simulink model "sampleModel2013"  (R2023a)
settings: Solver=VariableStepAuto  StartTime=0.0  StopTime=10.0  RelTol=1e-3
libraries: hdlsllib x3, simulink x1
settings Model: Creator=user1  LastModifiedBy=user1

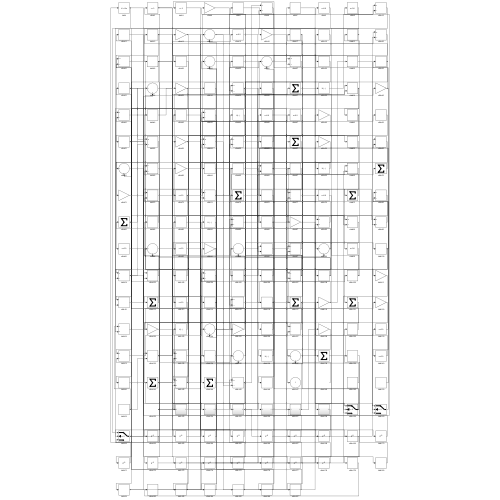
[thumbnail: Simulink's stored preview of the top-level diagram]
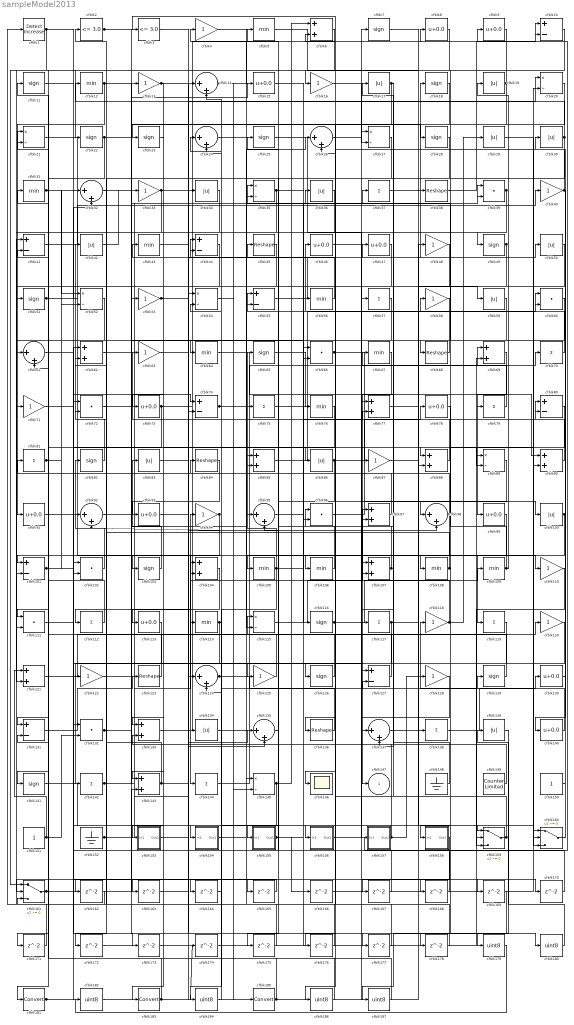
== system sampleModel2013 ==
  cfblk1 : simulink/Logic and Bit Operations/Detect Increase  vinit=0.0  OutDataTypeStr=boolean
      settings: LibrarySourceBlock=|
      | hdlsllib/Logic and Bit
      | Operations/Detect
      | Increase
  cfblk{10,41,44,55,74,80,101,127,131} (9 alike) : Sum  Inputs=+-
  cfblk{17,19,29..30,34,36,42,50,59,83,86,100,134,139} (14 alike) : Abs  SaturateOnIntegerOverflow=off
  cfblk{39,60,66,72,96,102,111,132} (8 alike) : DotProduct  OutDataTypeStr=Inherit: Inherit via internal rule
  cfblk{7,11,18,22..23,25,28,49,51,65,82,103,116,126,129,141} (16 alike) : Signum
  cfblk{6,62,69,77,85,88,90,97,104,107,121,133,143} (13 alike) : Sum
  cfblk{5,12,31,43,56,64,67,76,105..106,108..109,114} (13 alike) : MinMax
  cfblk{4,13,16,33,40,48,53,58,63,71,87,94,110,118,120,122,125,128} (18 alike) : Gain
  cfblk{37,57,70,75,79,81,112,117,119,138,142,144} (12 alike) : Sum  Inputs=+
  cfblk{8..9,15,46..47,73,78,91,93,99,113,130,140} (13 alike) : Bias  Bias=0.0  SaturateOnIntegerOverflow=off
  cfblk{20..21,27,35,52,54,89,115,145} (9 alike) : Product  Inputs=*/  RndMeth=Zero  SaturateOnIntegerOverflow=on
  cfblk{38,45,68,84,123,136} (6 alike) : Reshape
  cfblk{14,24,26,32,61,92,95,98,124,135,137} (11 alike) : Sum  Inputs=|++
  cfblk146 : Scope
  cfblk148 : Ground
  cfblk149 : hdlsllib/Sources/Counter Limited  uplimit=7  tsamp=-1
  cfblk150 : Constant  SampleTime=-1
  cfblk151 : Constant  SampleTime=-1
  cfblk152 : Ground
  cfblk153 : Subsystem
      settings: LibrarySourceBlock=|
      | hdlsllib/Ports &
      | Subsystems/Subsystem
  cfblk154 : Subsystem
      settings: LibrarySourceBlock=|
      | hdlsllib/Ports &
      | Subsystems/Subsystem
  cfblk155 : Subsystem
      settings: LibrarySourceBlock=|
      | hdlsllib/Ports &
      | Subsystems/Subsystem
  cfblk156 : Subsystem
      settings: LibrarySourceBlock=|
      | hdlsllib/Ports &
      | Subsystems/Subsystem
  cfblk157 : Subsystem
      settings: LibrarySourceBlock=|
      | hdlsllib/Ports &
      | Subsystems/Subsystem
  cfblk158 : Subsystem
      settings: LibrarySourceBlock=|
      | hdlsllib/Ports &
      | Subsystems/Subsystem
  cfblk159 : Switch  SaturateOnIntegerOverflow=off  InputSameDT=off
  cfblk160 : Switch  SaturateOnIntegerOverflow=off  InputSameDT=off
  cfblk161 : Switch  SaturateOnIntegerOverflow=off  InputSameDT=off
  cfblk{162..178} (17 alike) : Delay  SampleTime=1
  cfblk{179..180,182,184,186..187} (6 alike) : DataTypeConversion  OutDataTypeStr=uint8  SaturateOnIntegerOverflow=off  RndMeth=Floor
  cfblk181 : DataTypeConversion  SaturateOnIntegerOverflow=off  RndMeth=Floor
  cfblk183 : DataTypeConversion  SaturateOnIntegerOverflow=off  RndMeth=Floor
  cfblk185 : DataTypeConversion  SaturateOnIntegerOverflow=off  RndMeth=Floor
  cfblk2 : hdlsllib/Logic and Bit Operations/Compare To Constant  relop=<=  const=3.0  OutDataTypeStr=boolean
  cfblk3 : hdlsllib/Logic and Bit Operations/Compare To Constant  relop=<=  const=3.0  OutDataTypeStr=boolean
  cfblk147 : Outport  VectorParamsAs1DForOutWhenUnconnected=off
  wires:
  cfblk100/1 -> cfblk119/1, cfblk30/1, cfblk160/3
  cfblk42/1 -> cfblk33/1
  cfblk86/1 -> cfblk78/1, cfblk125/1
  cfblk160/1 -> cfblk80/1
  cfblk70/1 -> cfblk46/1
  cfblk141/1 -> cfblk156/1(In1)
  cfblk12/1 -> cfblk91/1, cfblk89/1
  cfblk73/1 -> cfblk45/1, cfblk101/1
  cfblk96/1 -> cfblk98/1
  cfblk140/1 -> cfblk118/1
  cfblk112/1 -> cfblk31/1
  cfblk142/1 -> cfblk37/1, cfblk120/1
  cfblk64/1 -> cfblk90/1
  cfblk135/1 -> cfblk5/1
  cfblk41/1 -> cfblk40/1
  cfblk144/1 -> cfblk69/1
  cfblk81/1 -> cfblk11/1, cfblk52/2
  cfblk40/1 -> cfblk3/1, cfblk140/1
  cfblk131/1 -> cfblk123/1
  cfblk55/1 -> cfblk18/1
  cfblk35/1 -> cfblk111/1, cfblk89/2
  cfblk66/1 -> cfblk100/1, cfblk26/2
  cfblk103/1 -> cfblk83/1
  cfblk105/1 -> cfblk65/1, cfblk124/2, cfblk77/2
  cfblk57/1 -> cfblk71/1
  cfblk123/1 -> cfblk21/1
  cfblk133/1 -> cfblk8/1
  cfblk76/1 -> cfblk113/1
  cfblk106/1 -> cfblk75/1
  cfblk31/1 -> cfblk131/1, cfblk52/1, cfblk173/1
  cfblk134/1 -> cfblk129/1
  cfblk49/1 -> cfblk107/2, cfblk186/1
  cfblk94/1 -> cfblk111/2, cfblk92/2
  cfblk151/1 -> cfblk121/1, cfblk132/2
  cfblk125/1 -> cfblk115/1
  cfblk156/1(Out1) -> cfblk9/1
  cfblk152/1 -> cfblk94/1, cfblk134/1
  cfblk7/1 -> cfblk138/1
  cfblk18/1 -> cfblk106/1
  cfblk21/1 -> cfblk103/1
  cfblk127/1 -> cfblk96/1
  cfblk118/1 -> cfblk24/1, cfblk29/1
  cfblk36/1 -> cfblk96/2
  cfblk68/1 -> cfblk64/1
  cfblk97/1 -> cfblk81/1
  cfblk93/1 -> cfblk47/1
  cfblk4/1 -> cfblk88/1
  cfblk10/1 -> cfblk141/1
  cfblk79/1 -> cfblk17/1
  cfblk91/1 -> cfblk110/1
  cfblk28/1 -> cfblk112/1
  cfblk1/1 -> cfblk161/1, cfblk159/3
  cfblk33/1 -> cfblk14/1, cfblk101/2
  cfblk32/1 -> cfblk15/1
  cfblk107/1 -> cfblk56/1, cfblk4/1
  cfblk54/1 -> cfblk185/1
  cfblk98/1 -> cfblk146/1, cfblk67/1, cfblk44/1
  cfblk148/1 -> cfblk55/1
  cfblk82/1 -> cfblk42/1
  cfblk19/1 -> cfblk16/1, cfblk77/1
  cfblk90/1 -> cfblk63/1
  cfblk75/1 -> cfblk58/1
  cfblk121/1 -> cfblk13/1
  cfblk67/1 -> cfblk147/1
  cfblk8/1 -> cfblk121/2
  cfblk26/1 -> cfblk7/1
  cfblk47/1 -> cfblk102/2
  cfblk5/1 -> cfblk38/1
  cfblk78/1 -> cfblk108/1
  cfblk51/1 -> cfblk144/1, cfblk32/2
  cfblk101/1 -> cfblk127/1, cfblk32/1
  cfblk20/1 -> cfblk23/1
  cfblk99/1 -> cfblk105/1
  cfblk30/1 -> cfblk12/1, cfblk175/1
  cfblk161/1 -> cfblk72/1, cfblk143/2
  cfblk39/1 -> cfblk49/1, cfblk61/2
  cfblk72/1 -> cfblk53/1
  cfblk58/1 -> cfblk93/1
  cfblk80/1 -> cfblk158/1(In1)
  cfblk13/1 -> cfblk153/1(In1), cfblk165/1
  cfblk95/1 -> cfblk39/1
  cfblk155/1(Out1) -> cfblk70/1, cfblk166/1
  cfblk102/1 -> cfblk82/1
  cfblk159/1 -> cfblk97/1, cfblk36/1
  cfblk46/1 -> cfblk90/2
  cfblk56/1 -> cfblk43/1
  cfblk23/1 -> cfblk143/1
  cfblk48/1 -> cfblk115/2
  cfblk62/1 -> cfblk114/1
  cfblk71/1 -> cfblk74/1
  cfblk38/1 -> cfblk10/1
  cfblk87/1 -> cfblk159/1
  cfblk34/1 -> cfblk181/1
  cfblk115/1 -> cfblk97/2
  cfblk92/1 -> cfblk154/1(In1)
  cfblk27/1 -> cfblk155/1(In1)
  cfblk69/1 -> cfblk99/1
  cfblk111/1 -> cfblk62/1
  cfblk14/1 -> cfblk10/2, cfblk145/2
  cfblk145/1 -> cfblk6/1, cfblk164/1
  cfblk85/1 -> cfblk27/1
  cfblk154/1(Out1) -> cfblk85/1
  cfblk50/1 -> cfblk133/1
  cfblk128/1 -> cfblk137/1
  cfblk6/1 -> cfblk22/1
  cfblk149/1 -> cfblk133/2
  cfblk143/1 -> cfblk92/1, cfblk135/1
  cfblk157/1(Out1) -> cfblk104/1, cfblk128/1
  cfblk84/1 -> cfblk183/1
  cfblk77/1 -> cfblk79/1
  cfblk59/1 -> cfblk107/1
  cfblk43/1 -> cfblk74/2
  cfblk130/1 -> cfblk60/1
  cfblk9/1 -> cfblk68/1
  cfblk132/1 -> cfblk95/1, cfblk39/2
  cfblk138/1 -> cfblk130/1
  cfblk65/1 -> cfblk76/1
  cfblk153/1(Out1) -> cfblk20/1
  cfblk74/1 -> cfblk50/1, cfblk26/1
  cfblk22/1 -> cfblk126/1, cfblk61/1, cfblk177/1
  cfblk116/1 -> cfblk109/1, cfblk136/1
  cfblk88/1 -> cfblk25/1
  cfblk25/1 -> cfblk157/1(In1)
  cfblk60/1 -> cfblk117/1
  cfblk63/1 -> cfblk98/2
  cfblk24/1 -> cfblk87/1
  cfblk2/1 -> cfblk28/1, cfblk66/2
  cfblk136/1 -> cfblk24/2
  cfblk61/1 -> cfblk86/1
  cfblk16/1 -> cfblk27/2
  cfblk150/1 -> cfblk80/2
  cfblk45/1 -> cfblk51/1
  cfblk114/1 -> cfblk142/1, cfblk44/2
  cfblk17/1 -> cfblk137/2, cfblk35/2
  cfblk15/1 -> cfblk116/1
  cfblk124/1 -> cfblk55/2, cfblk127/2
  cfblk137/1 -> cfblk60/2
  cfblk29/1 -> cfblk160/1
  cfblk129/1 -> cfblk104/2
  cfblk110/1 -> cfblk159/2
  cfblk126/1 -> cfblk41/2
  cfblk37/1 -> cfblk59/1
  cfblk109/1 -> cfblk19/1, cfblk35/1
  cfblk53/1 -> cfblk73/1, cfblk135/2
  cfblk108/1 -> cfblk2/1, cfblk85/2
  cfblk117/1 -> cfblk160/2, cfblk122/1
  cfblk113/1 -> cfblk162/1
  cfblk162/1 -> cfblk1/1
  cfblk44/1 -> cfblk163/1
  cfblk163/1 -> cfblk124/1
  cfblk164/1 -> cfblk14/2
  cfblk165/1 -> cfblk161/2
  cfblk166/1 -> cfblk20/2
  cfblk158/1(Out1) -> cfblk167/1
  cfblk167/1 -> cfblk72/2
  cfblk122/1 -> cfblk168/1
  cfblk168/1 -> cfblk102/1
  cfblk83/1 -> cfblk169/1
  cfblk11/1 -> cfblk170/1
  cfblk170/1 -> cfblk95/2
  cfblk52/1 -> cfblk171/1
  cfblk171/1 -> cfblk161/3
  cfblk104/1 -> cfblk172/1
  cfblk172/1 -> cfblk88/2
  cfblk173/1 -> cfblk69/2
  cfblk174/1 -> cfblk66/1
  cfblk175/1 -> cfblk41/1
  cfblk89/1 -> cfblk176/1
  cfblk176/1 -> cfblk145/1
  cfblk177/1 -> cfblk6/2
  cfblk120/1 -> cfblk178/1
  cfblk178/1 -> cfblk62/2
  cfblk139/1 -> cfblk179/1
  cfblk3/1 -> cfblk180/1
  cfblk180/1 -> cfblk139/1
  cfblk181/1 -> cfblk132/1, cfblk57/1
  cfblk179/1 -> cfblk182/1
  cfblk182/1 -> cfblk34/1
  cfblk183/1 -> cfblk174/1, cfblk21/2
  cfblk119/1 -> cfblk184/1
  cfblk184/1 -> cfblk84/1
  cfblk185/1 -> cfblk48/1, cfblk131/2
  cfblk186/1 -> cfblk54/1
  cfblk169/1 -> cfblk187/1
  cfblk187/1 -> cfblk54/2

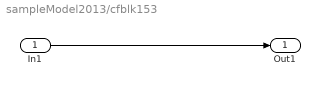
== system sampleModel2013/cfblk153 ==
  In1 : Inport
  Out1 : Outport
  wires:
  In1/1 -> Out1/1

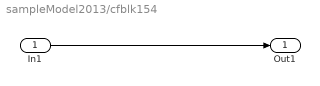
== system sampleModel2013/cfblk154 ==
  In1 : Inport
  Out1 : Outport
  wires:
  In1/1 -> Out1/1

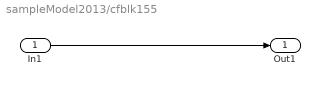
== system sampleModel2013/cfblk155 ==
  In1 : Inport
  Out1 : Outport
  wires:
  In1/1 -> Out1/1

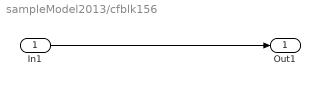
== system sampleModel2013/cfblk156 ==
  In1 : Inport
  Out1 : Outport
  wires:
  In1/1 -> Out1/1

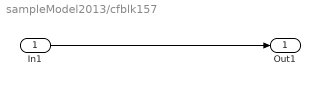
== system sampleModel2013/cfblk157 ==
  In1 : Inport
  Out1 : Outport
  wires:
  In1/1 -> Out1/1

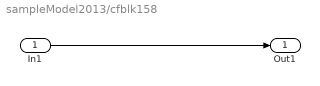
== system sampleModel2013/cfblk158 ==
  In1 : Inport
  Out1 : Outport
  wires:
  In1/1 -> Out1/1
